simulink model "TCMSSystem"  (R2019b)
settings: configuration reference "ConfigSet_TCMSSystem_Reference" (kept outside this file)
model workspace (MAT data in the model file):
  Prm_TCMSSystem : Simulink.Parameter (value not decoded)
  SampleTime = 0.05
symbols that are objects in the model workspace (value not decoded): Prm_TCMSSystem
undefined symbols (not defined in the file): ADDIntervention, AK1Status, AK2Status, AKContactorStatus, AllDoorsClosed, AllLeftDoorsClosed, AllRightDoorsClosed, APS1Fault, APS1Isolated, APS1OutputVoltage, APS1Status, APS2Fault, APS2Isolated, APS2OutputVoltage, APS2Status, APSKAKContactor, ASCOEnd1, ASCOEnd2, ATBMode, ATCBypassMode, ATCStatusNotOK, ATOMode, ATPLowSpeedCutoutStatus, ATPMode, AuxCompressor, BatteryCurrent, BatteryIsolationContactor, BatteryTemperature, BatteryVoltage, BCG1Fault, BCG1Isolated, BCG1IsolationFailed, BCG1OutputCurrent, BCG1Status, BCG2Fault, BCG2Isolated, BCG2OutputCurrent, BCG2Status, BCGOutputVoltage, BECU1AxleLockedWheelSet1, BECU2AxleLockedWheelSet2, BECUFaulty, BECUMajorFault, BECUMinorFault, BECUStatus, BIC1Inside, BIC1Outside, BIC2Inside, BIC2Outside, Bogie, Bogie1WSPStatus, Bogie2WSPStatus, BogieFaulty, BogieIsolationStatus, BogieSupportedMass, BrakeCylinderPressureGauge, BrakeLoopCBTripped, BrakeLoopOpenTL, BrakeTrainLineStatus, BrakingDemand ... (+215)
libraries: TimersLib x257, simulink x137, LatchesLib x42, VectorOperationsLib x15, TestBenchLib x12, MathOperationsLib x2, FiltersLib x1
(part 11 of 16)

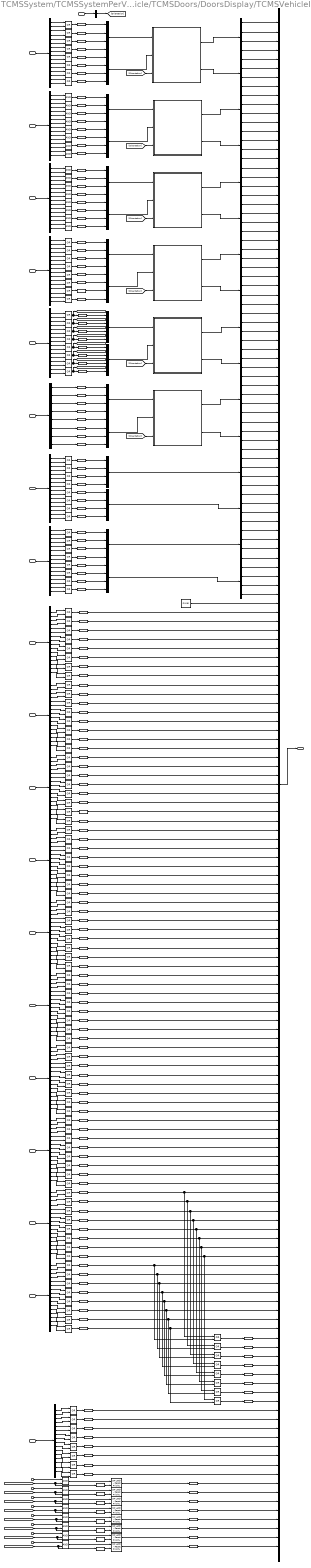
== system TCMSSystem/TCMSSystemPerVehicle/EnabledTCMSVehicle/TCMSDoors/DoorsDisplay/TCMSVehicleInfo/Subsystem1 ==
  CommonVehicleConfig : Inport
  DoorOpenStatus : Inport  Port=2
  DoorEmergencyReleasedStatus : Inport  Port=3
  DoorIsolatedStatus : Inport  Port=4
  DoorFaultStatus : Inport  Port=5
  DoorLockedStatus : Inport  Port=6
  DoorCloseObstruction : Inport  Port=7
  DoorOpenObstruction : Inport  Port=8
  DoorMotorCircuitFailure : Inport  Port=9
  DoorFailedToLock : Inport  Port=10
  DoorFailedToUnlock : Inport  Port=11
  DoorUnexpectedUnlocking : Inport  Port=12
  DCUFailure : Inport  Port=13
  DCSRFailure : Inport  Port=14
  DCSLFailure : Inport  Port=15
  DLSRFailure : Inport  Port=16
  DLSLFailure : Inport  Port=17
  DoorMajorFault : Inport  Port=18
  UnexpectedDoorOpeningDetectedByCC : Inport  Port=19
  DCUPower : Inport  Port=20
  In Bus Element : Inport  Port=21  PortName=InputControlStates  Element=LeftDoor1EED
  In Bus Element2 : Inport  Port=21  PortName=InputControlStates  Element=LeftDoor2EED
  In Bus Element3 : Inport  Port=21  PortName=InputControlStates  Element=LeftDoor3EED
  In Bus Element4 : Inport  Port=21  PortName=InputControlStates  Element=LeftDoor4EED
  In Bus Element5 : Inport  Port=21  PortName=InputControlStates  Element=RightDoor1EED
  In Bus Element6 : Inport  Port=21  PortName=InputControlStates  Element=RightDoor2EED
  In Bus Element7 : Inport  Port=21  PortName=InputControlStates  Element=RightDoor3EED
  In Bus Element8 : Inport  Port=21  PortName=InputControlStates  Element=RightDoor4EED
  Bus Creator : BusCreator  Inputs=169  OutDataTypeStr=Bus: BD_TCMSSystem_Out_Vehicle_Display_DoorSystem_Door  NonVirtualBus=on
  Bus Selector : BusSelector  OutputSignals=Orientation
  Data Type Conversion{1..168} (168 alike) : DataTypeConversion
  Demux : Demux  Outputs=8
  Demux{1..4,17,22,24..35} (18 alike) : Demux  Outputs=16
  Demux{5..16,19..21,23} (16 alike) : Demux
  Detect Decrease{,1..7} (8 alike) : simulink/Logic and Bit Operations/Detect Decrease  vinit=0.0  OutDataTypeStr=boolean
  FIXME2 : TestBenchLib/FIXME
      settings: SourceProductName=Sydac Utilities
  For Each Subsystem1 : Subsystem  TreatAsAtomicUnit=on
  For Each Subsystem2 : Subsystem  TreatAsAtomicUnit=on
  For Each Subsystem3 : Subsystem  TreatAsAtomicUnit=on
  For Each Subsystem4 : Subsystem  TreatAsAtomicUnit=on
  For Each Subsystem5 : Subsystem  TreatAsAtomicUnit=on
  For Each Subsystem6 : Subsystem  TreatAsAtomicUnit=on
  OR{,1..15,24..39,48..135,144..159} (136 alike) : Logic  Operator=OR  AllPortsSameDT=off  OutDataTypeStr=boolean
  OR{16..23,40..47,136..143} (24 alike) : Logic  AllPortsSameDT=off  OutDataTypeStr=boolean
  SR Latch - Reset Priority{,1..7} (8 alike) : LatchesLib/SR Latch - Reset Priority  initial_condition=0
      settings: SourceProductName=Latches
  Vector Concatenate{,1..15} (16 alike) : Concatenate  NumInputs=4
  TCMSDoorStatus : Outport
  wires:
  Bus Creator/1 -> TCMSDoorStatus/1
  Demux13/3 -> Bus Creator/39  "DoorB3EmergencyReleased"
  Demux14/4 -> Bus Creator/36  "DoorA4EmergencyReleased"
  Demux14/2 -> Bus Creator/34  "DoorA2EmergencyReleased"
  Demux13/2 -> Bus Creator/38  "DoorB2EmergencyReleased"
  Demux14/1 -> Bus Creator/33  "DoorA1EmergencyReleased"
  Demux13/1 -> Bus Creator/37  "DoorB1EmergencyReleased"
  Demux13/4 -> Bus Creator/40  "DoorB4EmergencyReleased"
  Demux14/3 -> Bus Creator/35  "DoorA3EmergencyReleased"
  Demux10/4 -> Bus Creator/24  "DoorB4Isolated"
  Demux10/3 -> Bus Creator/23  "DoorB3Isolated"
  Demux10/2 -> Bus Creator/22  "DoorB2Isolated"
  Demux10/1 -> Bus Creator/21  "DoorB1Isolated"
  Demux9/3 -> Bus Creator/19  "DoorA3Isolated"
  Demux9/4 -> Bus Creator/20  "DoorA4Isolated"
  Demux9/1 -> Bus Creator/17  "DoorA1Isolated"
  Demux9/2 -> Bus Creator/18  "DoorA2Isolated"
  Demux11/4 -> Bus Creator/32  "DoorB4Fault"
  Demux12/1 -> Bus Creator/25  "DoorA1Fault"
  Demux12/4 -> Bus Creator/28  "DoorA4Fault"
  Demux12/3 -> Bus Creator/27  "DoorA3Fault"
  Demux12/2 -> Bus Creator/26  "DoorA2Fault"
  Demux11/3 -> Bus Creator/31  "DoorB3Fault"
  Demux11/1 -> Bus Creator/29  "DoorB1Fault"
  Demux11/2 -> Bus Creator/30  "DoorB2Fault"
  CommonVehicleConfig/1 -> Bus Selector/1
  Demux7/1 -> Bus Creator/9  "DoorA1Locked"
  Demux7/2 -> Bus Creator/10  "DoorA2Locked"
  Demux7/3 -> Bus Creator/11  "DoorA3Locked"
  Demux7/4 -> Bus Creator/12  "DoorA4Locked"
  Demux8/1 -> Bus Creator/13  "DoorB1Locked"
  Demux8/2 -> Bus Creator/14  "DoorB2Locked"
  Demux8/3 -> Bus Creator/15  "DoorB3Locked"
  Demux8/4 -> Bus Creator/16  "DoorB4Locked"
  Demux5/1 -> Bus Creator/1  "DoorA1Open"
  Demux5/2 -> Bus Creator/2  "DoorA2Open"
  Demux5/3 -> Bus Creator/3  "DoorA3Open"
  Demux5/4 -> Bus Creator/4  "DoorA4Open"
  Demux6/1 -> Bus Creator/5  "DoorB1Open"
  Demux6/2 -> Bus Creator/6  "DoorB2Open"
  Demux6/3 -> Bus Creator/7  "DoorB3Open"
  Demux6/4 -> Bus Creator/8  "DoorB4Open"
  Data Type Conversion152/1 -> Vector Concatenate/1  "DoorA1Open"
  Data Type Conversion153/1 -> Vector Concatenate/2  "DoorA2Open"
  Data Type Conversion146/1 -> Vector Concatenate/3  "DoorA3Open"
  Data Type Conversion147/1 -> Vector Concatenate/4  "DoorA4Open"
  Data Type Conversion150/1 -> Vector Concatenate1/1  "DoorB1Open"
  Data Type Conversion151/1 -> Vector Concatenate1/2  "DoorB2Open"
  Data Type Conversion148/1 -> Vector Concatenate1/3  "DoorB3Open"
  Data Type Conversion149/1 -> Vector Concatenate1/4  "DoorB4Open"
  Bus Selector/1 -> [Orientation]  "<Orientation>"
  Data Type Conversion98/1 -> Vector Concatenate2/1  "DoorA1Locked"
  Data Type Conversion99/1 -> Vector Concatenate2/2  "DoorA2Locked"
  Data Type Conversion100/1 -> Vector Concatenate2/3  "DoorA3Locked"
  Data Type Conversion101/1 -> Vector Concatenate2/4  "DoorA4Locked"
  Data Type Conversion104/1 -> Vector Concatenate3/1  "DoorB1Locked"
  Data Type Conversion105/1 -> Vector Concatenate3/2  "DoorB2Locked"
  Data Type Conversion102/1 -> Vector Concatenate3/3  "DoorB3Locked"
  Data Type Conversion103/1 -> Vector Concatenate3/4  "DoorB4Locked"
  Data Type Conversion144/1 -> Vector Concatenate4/1  "DoorA1Isolated"
  Data Type Conversion145/1 -> Vector Concatenate4/2  "DoorA2Isolated"
  Data Type Conversion138/1 -> Vector Concatenate4/3  "DoorA3Isolated"
  Data Type Conversion139/1 -> Vector Concatenate4/4  "DoorA4Isolated"
  Data Type Conversion142/1 -> Vector Concatenate5/1  "DoorB1Isolated"
  Data Type Conversion143/1 -> Vector Concatenate5/2  "DoorB2Isolated"
  Data Type Conversion140/1 -> Vector Concatenate5/3  "DoorB3Isolated"
  Data Type Conversion141/1 -> Vector Concatenate5/4  "DoorB4Isolated"
  Data Type Conversion136/1 -> Vector Concatenate6/1  "DoorA1Fault"
  Data Type Conversion137/1 -> Vector Concatenate6/2  "DoorA2Fault"
  Data Type Conversion130/1 -> Vector Concatenate6/3  "DoorA3Fault"
  Data Type Conversion131/1 -> Vector Concatenate6/4  "DoorA4Fault"
  Data Type Conversion134/1 -> Vector Concatenate7/1  "DoorB1Fault"
  Data Type Conversion135/1 -> Vector Concatenate7/2  "DoorB2Fault"
  Data Type Conversion132/1 -> Vector Concatenate7/3  "DoorB3Fault"
  Data Type Conversion133/1 -> Vector Concatenate7/4  "DoorB4Fault"
  Data Type Conversion128/1 -> Vector Concatenate8/1  "DoorA1EmergencyReleased"
  Data Type Conversion129/1 -> Vector Concatenate8/2  "DoorA2EmergencyReleased"
  Data Type Conversion122/1 -> Vector Concatenate8/3  "DoorA3EmergencyReleased"
  Data Type Conversion123/1 -> Vector Concatenate8/4  "DoorA4EmergencyReleased"
  Data Type Conversion126/1 -> Vector Concatenate9/1  "DoorB1EmergencyReleased"
  Data Type Conversion127/1 -> Vector Concatenate9/2  "DoorB2EmergencyReleased"
  Data Type Conversion124/1 -> Vector Concatenate9/3  "DoorB3EmergencyReleased"
  Data Type Conversion125/1 -> Vector Concatenate9/4  "DoorB4EmergencyReleased"
  Demux16/3 -> Bus Creator/43  "DCU3Status"
  Demux15/4 -> Bus Creator/48  "DCU8Status"
  Demux15/1 -> Bus Creator/45  "DCU5Status"
  Demux15/2 -> Bus Creator/46  "DCU6Status"
  Demux16/2 -> Bus Creator/42  "DCU2Status"
  Demux16/4 -> Bus Creator/44  "DCU4Status"
  Demux15/3 -> Bus Creator/47  "DCU7Status"
  Demux16/1 -> Bus Creator/41  "DCU1Status"
  For Each Subsystem2/1(WireState1) -> Demux5/1
  For Each Subsystem2/2(WireState2) -> Demux6/1
  Vector Concatenate1/1 -> For Each Subsystem2/2(Source2)
  Vector Concatenate/1 -> For Each Subsystem2/1(Source1)
  [Orientation] -> For Each Subsystem2/3(Orientation)
  [Orientation] -> For Each Subsystem3/3(Orientation)
  Vector Concatenate2/1 -> For Each Subsystem3/1(Source1)
  Vector Concatenate3/1 -> For Each Subsystem3/2(Source2)
  For Each Subsystem3/2(WireState2) -> Demux8/1
  For Each Subsystem3/1(WireState1) -> Demux7/1
  For Each Subsystem4/1(WireState1) -> Demux9/1
  For Each Subsystem4/2(WireState2) -> Demux10/1
  Vector Concatenate5/1 -> For Each Subsystem4/2(Source2)
  Vector Concatenate4/1 -> For Each Subsystem4/1(Source1)
  [Orientation] -> For Each Subsystem4/3(Orientation)
  [Orientation] -> For Each Subsystem5/3(Orientation)
  Vector Concatenate8/1 -> For Each Subsystem5/1(Source1)
  Vector Concatenate9/1 -> For Each Subsystem5/2(Source2)
  For Each Subsystem5/2(WireState2) -> Demux13/1
  For Each Subsystem5/1(WireState1) -> Demux14/1
  [Orientation] -> For Each Subsystem1/3(Orientation)
  Vector Concatenate6/1 -> For Each Subsystem1/1(Source1)
  Vector Concatenate7/1 -> For Each Subsystem1/2(Source2)
  For Each Subsystem1/2(WireState2) -> Demux11/1
  For Each Subsystem1/1(WireState1) -> Demux12/1
  Data Type Conversion17/1 -> Bus Creator/73  "DoorB4MotorCircuitFailure"
  Data Type Conversion15/1 -> Bus Creator/71  "DoorB2MotorCircuitFailure"
  Data Type Conversion16/1 -> Bus Creator/72  "DoorB3MotorCircuitFailure"
  Demux21/4 -> Bus Creator/52  "DoorA4CloseObstruction"
  Vector Concatenate12/1 -> Demux23/1
  Vector Concatenate10/1 -> Demux21/1
  Vector Concatenate11/1 -> Demux20/1
  Demux23/2 -> Bus Creator/58  "DoorA2OpenObstruction"
  Data Type Conversion110/1 -> Vector Concatenate13/1  "DoorB1OpenObstruction"
  Demux19/3 -> Bus Creator/63  "DoorB3OpenObstruction"
  Data Type Conversion109/1 -> Vector Concatenate13/4  "DoorB4OpenObstruction"
  Data Type Conversion112/1 -> Vector Concatenate12/1  "DoorA1OpenObstruction"
  Data Type Conversion108/1 -> Vector Concatenate13/3  "DoorB3OpenObstruction"
  Demux19/1 -> Bus Creator/61  "DoorB1OpenObstruction"
  Data Type Conversion111/1 -> Vector Concatenate13/2  "DoorB2OpenObstruction"
  Data Type Conversion121/1 -> Vector Concatenate10/2  "DoorA2CloseObstruction"
  Demux21/1 -> Bus Creator/49  "DoorA1CloseObstruction"
  Data Type Conversion115/1 -> Vector Concatenate10/4  "DoorA4CloseObstruction"
  Demux21/2 -> Bus Creator/50  "DoorA2CloseObstruction"
  Demux20/2 -> Bus Creator/54  "DoorB2CloseObstruction"
  Demux21/3 -> Bus Creator/51  "DoorA3CloseObstruction"
  Demux23/1 -> Bus Creator/57  "DoorA1OpenObstruction"
  Data Type Conversion114/1 -> Vector Concatenate10/3  "DoorA3CloseObstruction"
  Vector Concatenate13/1 -> Demux19/1
  Data Type Conversion92/1 -> Bus Creator/76  "DoorA3FailedToLock"
  Data Type Conversion96/1 -> Bus Creator/80  "DoorB3FailedToLock"
  Data Type Conversion90/1 -> Bus Creator/74  "DoorA1FailedToLock"
  Data Type Conversion97/1 -> Bus Creator/81  "DoorB4FailedToLock"
  Data Type Conversion91/1 -> Bus Creator/75  "DoorA2FailedToLock"
  Data Type Conversion94/1 -> Bus Creator/78  "DoorB1FailedToLock"
  Data Type Conversion62/1 -> Bus Creator/110  "DoorB1DCSLFailure"
  Data Type Conversion95/1 -> Bus Creator/79  "DoorB2FailedToLock"
  Data Type Conversion60/1 -> Bus Creator/108  "DoorA3DCSLFailure"
  Data Type Conversion52/1 -> Bus Creator/116  "DoorA3DLSRFailure"
  Data Type Conversion50/1 -> Bus Creator/114  "DoorA1DLSRFailure"
  Data Type Conversion63/1 -> Bus Creator/111  "DoorB2DCSLFailure"
  Data Type Conversion51/1 -> Bus Creator/115  "DoorA2DLSRFailure"
  Data Type Conversion61/1 -> Bus Creator/109  "DoorA4DCSLFailure"
  Data Type Conversion65/1 -> Bus Creator/113  "DoorB4DCSLFailure"
  Data Type Conversion87/1 -> Bus Creator/87  "DoorB2FailedToUnlock"
  Data Type Conversion89/1 -> Bus Creator/89  "DoorB4FailedToUnlock"
  Data Type Conversion86/1 -> Bus Creator/86  "DoorB1FailedToUnlock"
  Data Type Conversion88/1 -> Bus Creator/88  "DoorB3FailedToUnlock"
  Data Type Conversion84/1 -> Bus Creator/84  "DoorA3FailedToUnlock"
  Data Type Conversion83/1 -> Bus Creator/83  "DoorA2FailedToUnlock"
  Data Type Conversion82/1 -> Bus Creator/82  "DoorA1FailedToUnlock"
  Data Type Conversion117/1 -> Vector Concatenate11/4  "DoorB4CloseObstruction"
  Data Type Conversion85/1 -> Bus Creator/85  "DoorA4FailedToUnlock"
  Data Type Conversion113/1 -> Vector Concatenate12/2  "DoorA2OpenObstruction"
  Data Type Conversion13/1 -> Bus Creator/69  "DoorA4MotorCircuitFailure"
  Data Type Conversion120/1 -> Vector Concatenate10/1  "DoorA1CloseObstruction"
  Data Type Conversion14/1 -> Bus Creator/70  "DoorB1MotorCircuitFailure"
  Data Type Conversion11/1 -> Bus Creator/67  "DoorA2MotorCircuitFailure"
  Demux20/4 -> Bus Creator/56  "DoorB4CloseObstruction"
  Data Type Conversion79/1 -> Bus Creator/95  "DoorB2UnexpectedUnlocking"
  Data Type Conversion75/1 -> Bus Creator/91  "DoorA2UnexpectedUnlocking"
  Data Type Conversion80/1 -> Bus Creator/96  "DoorB3UnexpectedUnlocking"
  Data Type Conversion119/1 -> Vector Concatenate11/2  "DoorB2CloseObstruction"
  Data Type Conversion78/1 -> Bus Creator/94  "DoorB1UnexpectedUnlocking"
  Data Type Conversion28/1 -> OR2/2, Bus Creator/140  "DoorA3DCUFailure"
  Data Type Conversion81/1 -> Bus Creator/97  "DoorB4UnexpectedUnlocking"
  Demux23/4 -> Bus Creator/60  "DoorA4OpenObstruction"
  Demux20/3 -> Bus Creator/55  "DoorB3CloseObstruction"
  Data Type Conversion106/1 -> Vector Concatenate12/3  "DoorA3OpenObstruction"
  Demux19/2 -> Bus Creator/62  "DoorB2OpenObstruction"
  Data Type Conversion26/1 -> OR/2, Bus Creator/138  "DoorA1DCUFailure"
  Data Type Conversion31/1 -> OR5/2, Bus Creator/143  "DoorB2DCUFailure"
  Data Type Conversion27/1 -> OR1/2, Bus Creator/139  "DoorA2DCUFailure"
  Data Type Conversion32/1 -> OR6/2, Bus Creator/144  "DoorB3DCUFailure"
  Data Type Conversion30/1 -> OR4/2, Bus Creator/142  "DoorB1DCUFailure"
  Data Type Conversion54/1 -> Bus Creator/118  "DoorB1DLSRFailure"
  Data Type Conversion34/1 -> OR/1, Bus Creator/130  "DoorA1DoorMajorFault"
  Data Type Conversion56/1 -> Bus Creator/120  "DoorB3DLSRFailure"
  Data Type Conversion107/1 -> Vector Concatenate12/4  "DoorA4OpenObstruction"
  Data Type Conversion40/1 -> OR6/1, Bus Creator/136  "DoorB3DoorMajorFault"
  Data Type Conversion76/1 -> Bus Creator/92  "DoorA3UnexpectedUnlocking"
  Data Type Conversion58/1 -> Bus Creator/106  "DoorA1DCSLFailure"
  Data Type Conversion53/1 -> Bus Creator/117  "DoorA4DLSRFailure"
  Data Type Conversion33/1 -> OR7/2, Bus Creator/145  "DoorB4DCUFailure"
  Data Type Conversion72/1 -> Bus Creator/104  "DoorB3DCSRFailure"
  Data Type Conversion93/1 -> Bus Creator/77  "DoorA4FailedToLock"
  Data Type Conversion64/1 -> Bus Creator/112  "DoorB3DCSLFailure"
  Data Type Conversion71/1 -> Bus Creator/103  "DoorB2DCSRFailure"
  Data Type Conversion70/1 -> Bus Creator/102  "DoorB1DCSRFailure"
  Data Type Conversion74/1 -> Bus Creator/90  "DoorA1UnexpectedUnlocking"
  Data Type Conversion73/1 -> Bus Creator/105  "DoorB4DCSRFailure"
  Demux23/3 -> Bus Creator/59  "DoorA3OpenObstruction"
  Data Type Conversion68/1 -> Bus Creator/100  "DoorA3DCSRFailure"
  Data Type Conversion12/1 -> Bus Creator/68  "DoorA3MotorCircuitFailure"
  Data Type Conversion67/1 -> Bus Creator/99  "DoorA2DCSRFailure"
  Data Type Conversion66/1 -> Bus Creator/98  "DoorA1DCSRFailure"
  Data Type Conversion38/1 -> OR4/1, Bus Creator/134  "DoorB1DoorMajorFault"
  Data Type Conversion44/1 -> Bus Creator/124  "DoorA3DLSLFailure"
  Data Type Conversion48/1 -> Bus Creator/128  "DoorB3DLSLFailure"
  FIXME2/1 -> Bus Creator/65  "DoorA1OpenDummyForLeaf"
  Data Type Conversion35/1 -> OR1/1, Bus Creator/131  "DoorA2DoorMajorFault"
  Data Type Conversion10/1 -> Bus Creator/66  "DoorA1MotorCircuitFailure"
  Data Type Conversion45/1 -> Bus Creator/125  "DoorA4DLSLFailure"
  Data Type Conversion118/1 -> Vector Concatenate11/1  "DoorB1CloseObstruction"
  Data Type Conversion46/1 -> Bus Creator/126  "DoorB1DLSLFailure"
  Demux19/4 -> Bus Creator/64  "DoorB4OpenObstruction"
  Data Type Conversion55/1 -> Bus Creator/119  "DoorB2DLSRFailure"
  Data Type Conversion37/1 -> OR3/1, Bus Creator/133  "DoorA4DoorMajorFault"
  Demux20/1 -> Bus Creator/53  "DoorB1CloseObstruction"
  Data Type Conversion49/1 -> Bus Creator/129  "DoorB4DLSLFailure"
  Data Type Conversion43/1 -> Bus Creator/123  "DoorA2DLSLFailure"
  Data Type Conversion42/1 -> Bus Creator/122  "DoorA1DLSLFailure"
  Data Type Conversion69/1 -> Bus Creator/101  "DoorA4DCSRFailure"
  Data Type Conversion36/1 -> OR2/1, Bus Creator/132  "DoorA3DoorMajorFault"
  Data Type Conversion59/1 -> Bus Creator/107  "DoorA2DCSLFailure"
  Data Type Conversion39/1 -> OR5/1, Bus Creator/135  "DoorB2DoorMajorFault"
  Data Type Conversion41/1 -> OR7/1, Bus Creator/137  "DoorB4DoorMajorFault"
  Data Type Conversion77/1 -> Bus Creator/93  "DoorA4UnexpectedUnlocking"
  Data Type Conversion47/1 -> Bus Creator/127  "DoorB2DLSLFailure"
  Data Type Conversion29/1 -> OR3/2, Bus Creator/141  "DoorA4DCUFailure"
  Data Type Conversion116/1 -> Vector Concatenate11/3  "DoorB3CloseObstruction"
  Data Type Conversion57/1 -> Bus Creator/121  "DoorB4DLSRFailure"
  OR2/1 -> Data Type Conversion4/1
  OR/1 -> Data Type Conversion2/1
  OR6/1 -> Data Type Conversion8/1
  OR1/1 -> Data Type Conversion3/1
  OR4/1 -> Data Type Conversion6/1
  OR3/1 -> Data Type Conversion5/1
  OR7/1 -> Data Type Conversion9/1
  OR5/1 -> Data Type Conversion7/1
  Data Type Conversion2/1 -> Bus Creator/146  "DCU1Fault"
  Data Type Conversion3/1 -> Bus Creator/147  "DCU2Fault"
  Data Type Conversion4/1 -> Bus Creator/148  "DCU3Fault"
  Data Type Conversion5/1 -> Bus Creator/149  "DCU4Fault"
  Data Type Conversion6/1 -> Bus Creator/150  "DCU5Fault"
  Data Type Conversion7/1 -> Bus Creator/151  "DCU6Fault"
  Data Type Conversion8/1 -> Bus Creator/152  "DCU7Fault"
  Data Type Conversion9/1 -> Bus Creator/153  "DCU8Fault"
  Data Type Conversion18/1 -> Bus Creator/154  "DoorA1UnexpectedOpen"
  Data Type Conversion19/1 -> Bus Creator/155  "DoorA2UnexpectedOpen"
  Data Type Conversion20/1 -> Bus Creator/156  "DoorA3UnexpectedOpen"
  Data Type Conversion21/1 -> Bus Creator/157  "DoorA4UnexpectedOpen"
  Data Type Conversion22/1 -> Bus Creator/158  "DoorB1UnexpectedOpen"
  Data Type Conversion23/1 -> Bus Creator/159  "DoorB2UnexpectedOpen"
  Data Type Conversion24/1 -> Bus Creator/160  "DoorB3UnexpectedOpen"
  Data Type Conversion25/1 -> Bus Creator/161  "DoorB4UnexpectedOpen"
  UnexpectedDoorOpeningDetectedByCC/1 -> Demux34/1  "DCU8Fault"
  Demux35/8 -> OR157/2
  Demux35/4 -> OR155/2
  Demux35/2 -> OR154/2
  Demux35/3 -> OR155/1
  Demux35/16 -> OR159/2
  Demux35/12 -> OR153/2
  Demux35/6 -> OR156/2
  Demux35/9 -> OR152/1
  Demux35/10 -> OR152/2
  Demux35/15 -> OR159/1
  Demux35/1 -> OR154/1
  Demux35/11 -> OR153/1
  Demux35/7 -> OR157/1
  Demux35/13 -> OR158/1
  Demux35/5 -> OR156/1
  Demux35/14 -> OR158/2
  OR154/1 -> Data Type Conversion10/1
  OR155/1 -> Data Type Conversion11/1
  OR157/1 -> Data Type Conversion13/1
  OR156/1 -> Data Type Conversion12/1
  OR158/1 -> Data Type Conversion16/1
  OR159/1 -> Data Type Conversion17/1
  OR153/1 -> Data Type Conversion15/1
  OR152/1 -> Data Type Conversion14/1
  OR144/1 -> Data Type Conversion22/1
  OR145/1 -> Data Type Conversion23/1
  OR151/1 -> Data Type Conversion25/1
  OR150/1 -> Data Type Conversion24/1
  OR148/1 -> Data Type Conversion20/1
  OR149/1 -> Data Type Conversion21/1
  OR147/1 -> Data Type Conversion19/1
  OR146/1 -> Data Type Conversion18/1
  Demux34/14 -> OR150/2
  Demux34/5 -> OR148/1
  Demux34/13 -> OR150/1
  Demux34/7 -> OR149/1
  Demux34/11 -> OR145/1
  Demux34/1 -> OR146/1
  Demux34/15 -> OR151/1
  Demux34/10 -> OR144/2
  Demux34/9 -> OR144/1
  Demux34/6 -> OR148/2
  Demux34/12 -> OR145/2
  Demux34/16 -> OR151/2
  Demux34/3 -> OR147/1
  Demux34/2 -> OR146/2
  Demux34/4 -> OR147/2
  Demux34/8 -> OR149/2
  OR64/1 -> Data Type Conversion30/1
  OR65/1 -> Data Type Conversion31/1
  OR71/1 -> Data Type Conversion33/1
  OR70/1 -> Data Type Conversion32/1
  OR68/1 -> Data Type Conversion28/1
  OR69/1 -> Data Type Conversion29/1
  OR67/1 -> Data Type Conversion27/1
  OR66/1 -> Data Type Conversion26/1
  Demux17/14 -> OR70/2
  Demux17/5 -> OR68/1
  Demux17/13 -> OR70/1
  Demux17/7 -> OR69/1
  Demux17/11 -> OR65/1
  Demux17/1 -> OR66/1
  Demux17/15 -> OR71/1
  Demux17/10 -> OR64/2
  Demux17/9 -> OR64/1
  Demux17/6 -> OR68/2
  Demux17/12 -> OR65/2
  Demux17/16 -> OR71/2
  Demux17/3 -> OR67/1
  Demux17/2 -> OR66/2
  Demux17/4 -> OR67/2
  Demux17/8 -> OR69/2
  DCUFailure/1 -> Demux17/1
  OR72/1 -> Data Type Conversion38/1
  OR73/1 -> Data Type Conversion39/1
  OR79/1 -> Data Type Conversion41/1
  OR78/1 -> Data Type Conversion40/1
  OR76/1 -> Data Type Conversion36/1
  OR77/1 -> Data Type Conversion37/1
  OR75/1 -> Data Type Conversion35/1
  OR74/1 -> Data Type Conversion34/1
  Demux25/14 -> OR78/2
  Demux25/5 -> OR76/1
  Demux25/13 -> OR78/1
  Demux25/7 -> OR77/1
  Demux25/11 -> OR73/1
  Demux25/1 -> OR74/1
  Demux25/15 -> OR79/1
  Demux25/10 -> OR72/2
  Demux25/9 -> OR72/1
  Demux25/6 -> OR76/2
  Demux25/12 -> OR73/2
  Demux25/16 -> OR79/2
  Demux25/3 -> OR75/1
  Demux25/2 -> OR74/2
  Demux25/4 -> OR75/2
  Demux25/8 -> OR77/2
  DoorMajorFault/1 -> Demux25/1
  OR80/1 -> Data Type Conversion46/1
  OR81/1 -> Data Type Conversion47/1
  OR87/1 -> Data Type Conversion49/1
  OR86/1 -> Data Type Conversion48/1
  OR84/1 -> Data Type Conversion44/1
  OR85/1 -> Data Type Conversion45/1
  OR83/1 -> Data Type Conversion43/1
  OR82/1 -> Data Type Conversion42/1
  Demux26/14 -> OR86/2
  Demux26/5 -> OR84/1
  Demux26/13 -> OR86/1
  Demux26/7 -> OR85/1
  Demux26/11 -> OR81/1
  Demux26/1 -> OR82/1
  Demux26/15 -> OR87/1
  Demux26/10 -> OR80/2
  Demux26/9 -> OR80/1
  Demux26/6 -> OR84/2
  Demux26/12 -> OR81/2
  Demux26/16 -> OR87/2
  Demux26/3 -> OR83/1
  Demux26/2 -> OR82/2
  Demux26/4 -> OR83/2
  Demux26/8 -> OR85/2
  DLSLFailure/1 -> Demux26/1
  OR88/1 -> Data Type Conversion54/1
  OR89/1 -> Data Type Conversion55/1
  OR95/1 -> Data Type Conversion57/1
  OR94/1 -> Data Type Conversion56/1
  OR92/1 -> Data Type Conversion52/1
  OR93/1 -> Data Type Conversion53/1
  OR91/1 -> Data Type Conversion51/1
  OR90/1 -> Data Type Conversion50/1
  Demux27/14 -> OR94/2
  Demux27/5 -> OR92/1
  Demux27/13 -> OR94/1
  Demux27/7 -> OR93/1
  Demux27/11 -> OR89/1
  Demux27/1 -> OR90/1
  Demux27/15 -> OR95/1
  Demux27/10 -> OR88/2
  Demux27/9 -> OR88/1
  Demux27/6 -> OR92/2
  Demux27/12 -> OR89/2
  Demux27/16 -> OR95/2
  Demux27/3 -> OR91/1
  Demux27/2 -> OR90/2
  Demux27/4 -> OR91/2
  Demux27/8 -> OR93/2
  DLSRFailure/1 -> Demux27/1
  OR96/1 -> Data Type Conversion62/1
  OR97/1 -> Data Type Conversion63/1
  OR103/1 -> Data Type Conversion65/1
  OR102/1 -> Data Type Conversion64/1
  OR100/1 -> Data Type Conversion60/1
  OR101/1 -> Data Type Conversion61/1
  OR99/1 -> Data Type Conversion59/1
  OR98/1 -> Data Type Conversion58/1
  Demux28/14 -> OR102/2
  Demux28/5 -> OR100/1
  Demux28/13 -> OR102/1
  Demux28/7 -> OR101/1
  Demux28/11 -> OR97/1
  Demux28/1 -> OR98/1
  Demux28/15 -> OR103/1
  Demux28/10 -> OR96/2
  Demux28/9 -> OR96/1
  Demux28/6 -> OR100/2
  Demux28/12 -> OR97/2
  Demux28/16 -> OR103/2
  Demux28/3 -> OR99/1
  Demux28/2 -> OR98/2
  Demux28/4 -> OR99/2
  Demux28/8 -> OR101/2
  DCSLFailure/1 -> Demux28/1
  OR104/1 -> Data Type Conversion70/1
  OR105/1 -> Data Type Conversion71/1
  OR111/1 -> Data Type Conversion73/1
  OR110/1 -> Data Type Conversion72/1
  OR108/1 -> Data Type Conversion68/1
  OR109/1 -> Data Type Conversion69/1
  OR107/1 -> Data Type Conversion67/1
  OR106/1 -> Data Type Conversion66/1
  Demux29/14 -> OR110/2
  Demux29/5 -> OR108/1
  Demux29/13 -> OR110/1
  Demux29/7 -> OR109/1
  Demux29/11 -> OR105/1
  Demux29/1 -> OR106/1
  Demux29/15 -> OR111/1
  Demux29/10 -> OR104/2
  Demux29/9 -> OR104/1
  Demux29/6 -> OR108/2
  Demux29/12 -> OR105/2
  Demux29/16 -> OR111/2
  Demux29/3 -> OR107/1
  Demux29/2 -> OR106/2
  Demux29/4 -> OR107/2
  Demux29/8 -> OR109/2
  OR112/1 -> Data Type Conversion78/1
  OR113/1 -> Data Type Conversion79/1
  OR119/1 -> Data Type Conversion81/1
  OR118/1 -> Data Type Conversion80/1
  OR116/1 -> Data Type Conversion76/1
  OR117/1 -> Data Type Conversion77/1
  OR115/1 -> Data Type Conversion75/1
  OR114/1 -> Data Type Conversion74/1
  Demux30/14 -> OR118/2
  Demux30/5 -> OR116/1
  Demux30/13 -> OR118/1
  Demux30/7 -> OR117/1
  Demux30/11 -> OR113/1
  Demux30/1 -> OR114/1
  Demux30/15 -> OR119/1
  Demux30/10 -> OR112/2
  Demux30/9 -> OR112/1
  Demux30/6 -> OR116/2
  Demux30/12 -> OR113/2
  Demux30/16 -> OR119/2
  Demux30/3 -> OR115/1
  Demux30/2 -> OR114/2
  Demux30/4 -> OR115/2
  Demux30/8 -> OR117/2
  OR120/1 -> Data Type Conversion86/1
  OR121/1 -> Data Type Conversion87/1
  OR127/1 -> Data Type Conversion89/1
  OR126/1 -> Data Type Conversion88/1
  OR124/1 -> Data Type Conversion84/1
  OR125/1 -> Data Type Conversion85/1
  OR123/1 -> Data Type Conversion83/1
  OR122/1 -> Data Type Conversion82/1
  Demux31/14 -> OR126/2
  Demux31/5 -> OR124/1
  Demux31/13 -> OR126/1
  Demux31/7 -> OR125/1
  Demux31/11 -> OR121/1
  Demux31/1 -> OR122/1
  Demux31/15 -> OR127/1
  Demux31/10 -> OR120/2
  Demux31/9 -> OR120/1
  Demux31/6 -> OR124/2
  Demux31/12 -> OR121/2
  Demux31/16 -> OR127/2
  Demux31/3 -> OR123/1
  Demux31/2 -> OR122/2
  Demux31/4 -> OR123/2
  Demux31/8 -> OR125/2
  OR128/1 -> Data Type Conversion94/1
  OR129/1 -> Data Type Conversion95/1
  OR135/1 -> Data Type Conversion97/1
  OR134/1 -> Data Type Conversion96/1
  OR132/1 -> Data Type Conversion92/1
  OR133/1 -> Data Type Conversion93/1
  OR131/1 -> Data Type Conversion91/1
  OR130/1 -> Data Type Conversion90/1
  Demux32/14 -> OR134/2
  Demux32/5 -> OR132/1
  Demux32/13 -> OR134/1
  Demux32/7 -> OR133/1
  Demux32/11 -> OR129/1
  Demux32/1 -> OR130/1
  Demux32/15 -> OR135/1
  Demux32/10 -> OR128/2
  Demux32/9 -> OR128/1
  Demux32/6 -> OR132/2
  Demux32/12 -> OR129/2
  Demux32/16 -> OR135/2
  Demux32/3 -> OR131/1
  Demux32/2 -> OR130/2
  Demux32/4 -> OR131/2
  Demux32/8 -> OR133/2
  DoorMotorCircuitFailure/1 -> Demux35/1
  DoorFailedToLock/1 -> Demux32/1
  DoorFailedToUnlock/1 -> Demux31/1
  DoorUnexpectedUnlocking/1 -> Demux30/1
  DCSRFailure/1 -> Demux29/1
  Demux33/14 -> OR18/2
  Demux33/5 -> OR16/1
  Demux33/13 -> OR18/1
  Demux33/7 -> OR17/1
  Demux33/11 -> OR21/1
  Demux33/1 -> OR22/1
  Demux33/15 -> OR19/1
  Demux33/10 -> OR20/2
  Demux33/9 -> OR20/1
  Demux33/6 -> OR16/2
  Demux33/12 -> OR21/2
  Demux33/16 -> OR19/2
  Demux33/3 -> OR23/1
  Demux33/2 -> OR22/2
  Demux33/4 -> OR23/2
  Demux33/8 -> OR17/2
  DoorLockedStatus/1 -> Demux33/1
  OR22/1 -> Data Type Conversion98/1
  OR23/1 -> Data Type Conversion99/1
  OR17/1 -> Data Type Conversion101/1
  OR16/1 -> Data Type Conversion100/1
  OR18/1 -> Data Type Conversion102/1
  OR19/1 -> Data Type Conversion103/1
  OR21/1 -> Data Type Conversion105/1
  OR20/1 -> Data Type Conversion104/1
  OR60/1 -> Data Type Conversion110/1
  OR61/1 -> Data Type Conversion111/1
  OR59/1 -> Data Type Conversion109/1
  OR58/1 -> Data Type Conversion108/1
  OR56/1 -> Data Type Conversion106/1
  OR57/1 -> Data Type Conversion107/1
  OR63/1 -> Data Type Conversion113/1
  OR62/1 -> Data Type Conversion112/1
  DoorOpenObstruction/1 -> Demux24/1
  Demux24/8 -> OR57/2
  Demux24/4 -> OR63/2
  Demux24/2 -> OR62/2
  Demux24/3 -> OR63/1
  Demux24/16 -> OR59/2
  Demux24/12 -> OR61/2
  Demux24/6 -> OR56/2
  Demux24/9 -> OR60/1
  Demux24/10 -> OR60/2
  Demux24/15 -> OR59/1
  Demux24/1 -> OR62/1
  Demux24/11 -> OR61/1
  Demux24/7 -> OR57/1
  Demux24/13 -> OR58/1
  Demux24/5 -> OR56/1
  Demux24/14 -> OR58/2
  OR52/1 -> Data Type Conversion118/1
  OR53/1 -> Data Type Conversion119/1
  OR51/1 -> Data Type Conversion117/1
  OR50/1 -> Data Type Conversion116/1
  OR48/1 -> Data Type Conversion114/1
  OR49/1 -> Data Type Conversion115/1
  OR55/1 -> Data Type Conversion121/1
  OR54/1 -> Data Type Conversion120/1
  DoorCloseObstruction/1 -> Demux22/1
  Demux22/8 -> OR49/2
  Demux22/4 -> OR55/2
  Demux22/2 -> OR54/2
  Demux22/3 -> OR55/1
  Demux22/16 -> OR51/2
  Demux22/12 -> OR53/2
  Demux22/6 -> OR48/2
  Demux22/9 -> OR52/1
  Demux22/10 -> OR52/2
  Demux22/15 -> OR51/1
  Demux22/1 -> OR54/1
  Demux22/11 -> OR53/1
  Demux22/7 -> OR49/1
  Demux22/13 -> OR50/1
  Demux22/5 -> OR48/1
  Demux22/14 -> OR50/2
  OR28/1 -> [DoorB1EmergencyReleased], Data Type Conversion126/1
  OR29/1 -> [DoorB2EmergencyReleased], Data Type Conversion127/1
  OR27/1 -> [DoorB4EmergencyReleased], Data Type Conversion125/1
  OR26/1 -> [DoorB3EmergencyReleased], Data Type Conversion124/1
  OR24/1 -> [DoorA3EmergencyReleased], Data Type Conversion122/1
  OR25/1 -> [DoorA4EmergencyReleased], Data Type Conversion123/1
  OR30/1 -> [DoorA1EmergencyReleased], Data Type Conversion128/1
  DoorEmergencyReleasedStatus/1 -> Demux2/1
  Demux2/8 -> OR25/2
  Demux2/4 -> OR31/2
  Demux2/2 -> OR30/2
  Demux2/3 -> OR31/1
  Demux2/16 -> OR27/2
  Demux2/12 -> OR29/2
  Demux2/6 -> OR24/2
  Demux2/9 -> OR28/1
  Demux2/10 -> OR28/2
  Demux2/15 -> OR27/1
  Demux2/1 -> OR30/1
  Demux2/11 -> OR29/1
  Demux2/7 -> OR25/1
  Demux2/13 -> OR26/1
  Demux2/5 -> OR24/1
  Demux2/14 -> OR26/2
  OR36/1 -> Data Type Conversion134/1
  OR37/1 -> Data Type Conversion135/1
  OR35/1 -> Data Type Conversion133/1
  OR34/1 -> Data Type Conversion132/1
  OR32/1 -> Data Type Conversion130/1
  OR33/1 -> Data Type Conversion131/1
  OR39/1 -> Data Type Conversion137/1
  OR38/1 -> Data Type Conversion136/1
  DoorFaultStatus/1 -> Demux3/1
  Demux3/8 -> OR33/2
  Demux3/4 -> OR39/2
  Demux3/2 -> OR38/2
  Demux3/3 -> OR39/1
  Demux3/16 -> OR35/2
  Demux3/12 -> OR37/2
  Demux3/6 -> OR32/2
  Demux3/9 -> OR36/1
  Demux3/10 -> OR36/2
  Demux3/15 -> OR35/1
  Demux3/1 -> OR38/1
  Demux3/11 -> OR37/1
  Demux3/7 -> OR33/1
  Demux3/13 -> OR34/1
  Demux3/5 -> OR32/1
  Demux3/14 -> OR34/2
  OR44/1 -> Data Type Conversion142/1
  OR45/1 -> Data Type Conversion143/1
  OR43/1 -> Data Type Conversion141/1
  OR42/1 -> Data Type Conversion140/1
  OR40/1 -> Data Type Conversion138/1
  OR41/1 -> Data Type Conversion139/1
  OR47/1 -> Data Type Conversion145/1
  OR46/1 -> Data Type Conversion144/1
  DoorIsolatedStatus/1 -> Demux4/1
  Demux4/8 -> OR41/2
  Demux4/4 -> OR47/2
  Demux4/2 -> OR46/2
  Demux4/3 -> OR47/1
  Demux4/16 -> OR43/2
  Demux4/12 -> OR45/2
  Demux4/6 -> OR40/2
  Demux4/9 -> OR44/1
  Demux4/10 -> OR44/2
  Demux4/15 -> OR43/1
  Demux4/1 -> OR46/1
  Demux4/11 -> OR45/1
  Demux4/7 -> OR41/1
  Demux4/13 -> OR42/1
  Demux4/5 -> OR40/1
  Demux4/14 -> OR42/2
  OR12/1 -> Data Type Conversion150/1
  OR13/1 -> Data Type Conversion151/1
  OR11/1 -> Data Type Conversion149/1
  OR10/1 -> Data Type Conversion148/1
  OR8/1 -> Data Type Conversion146/1
  OR9/1 -> Data Type Conversion147/1
  OR15/1 -> Data Type Conversion153/1
  OR14/1 -> Data Type Conversion152/1
  DoorOpenStatus/1 -> Demux1/1
  Demux1/8 -> OR9/2
  Demux1/4 -> OR15/2
  Demux1/2 -> OR14/2
  Demux1/3 -> OR15/1
  Demux1/16 -> OR11/2
  Demux1/12 -> OR13/2
  Demux1/6 -> OR8/2
  Demux1/9 -> OR12/1
  Demux1/10 -> OR12/2
  Demux1/15 -> OR11/1
  Demux1/1 -> OR14/1
  Demux1/11 -> OR13/1
  Demux1/7 -> OR9/1
  Demux1/13 -> OR10/1
  Demux1/5 -> OR8/1
  Demux1/14 -> OR10/2
  For Each Subsystem6/1(WireState1) -> Demux16/1
  For Each Subsystem6/2(WireState2) -> Demux15/1
  Vector Concatenate15/1 -> For Each Subsystem6/2(Source2)
  Vector Concatenate14/1 -> For Each Subsystem6/1(Source1)
  [Orientation] -> For Each Subsystem6/3(Orientation)
  Demux/1 -> Data Type Conversion1/1
  Demux/2 -> Data Type Conversion154/1
  Demux/3 -> Data Type Conversion155/1
  Demux/4 -> Data Type Conversion156/1
  Demux/5 -> Data Type Conversion157/1
  Demux/6 -> Data Type Conversion158/1
  Demux/7 -> Data Type Conversion159/1
  Demux/8 -> Data Type Conversion160/1
  DCUPower/1 -> Demux/1
  Data Type Conversion1/1 -> Vector Concatenate14/1
  Data Type Conversion154/1 -> Vector Concatenate14/2
  Data Type Conversion155/1 -> Vector Concatenate14/3
  Data Type Conversion156/1 -> Vector Concatenate14/4
  Data Type Conversion157/1 -> Vector Concatenate15/1
  Data Type Conversion158/1 -> Vector Concatenate15/2
  Data Type Conversion159/1 -> Vector Concatenate15/3
  Data Type Conversion160/1 -> Vector Concatenate15/4
  In Bus Element/1 -> OR142/1
  In Bus Element2/1 -> OR143/1
  In Bus Element3/1 -> OR136/1
  In Bus Element4/1 -> OR137/1
  In Bus Element5/1 -> OR140/1
  In Bus Element6/1 -> OR141/1
  In Bus Element7/1 -> OR138/1
  In Bus Element8/1 -> OR139/1
  OR142/1 -> SR Latch - Reset Priority/1
  OR143/1 -> SR Latch - Reset Priority1/1
  OR136/1 -> SR Latch - Reset Priority2/1
  OR137/1 -> SR Latch - Reset Priority3/1
  OR140/1 -> SR Latch - Reset Priority4/1
  OR141/1 -> SR Latch - Reset Priority5/1
  OR138/1 -> SR Latch - Reset Priority6/1
  OR139/1 -> SR Latch - Reset Priority7/1
  OR31/1 -> [DoorA2EmergencyReleased], Data Type Conversion129/1
  [DoorA4EmergencyReleased] -> Detect Decrease/1, OR137/2
  Detect Decrease/1 -> SR Latch - Reset Priority3/2
  Detect Decrease7/1 -> SR Latch - Reset Priority7/2
  Detect Decrease6/1 -> SR Latch - Reset Priority6/2
  Detect Decrease5/1 -> SR Latch - Reset Priority5/2
  Detect Decrease4/1 -> SR Latch - Reset Priority4/2
  [DoorA3EmergencyReleased] -> Detect Decrease1/1, OR136/2
  [DoorA2EmergencyReleased] -> Detect Decrease2/1, OR143/2
  [DoorA1EmergencyReleased] -> Detect Decrease3/1, OR142/2
  [DoorB1EmergencyReleased] -> Detect Decrease4/1, OR140/2
  [DoorB2EmergencyReleased] -> Detect Decrease5/1, OR141/2
  [DoorB3EmergencyReleased] -> Detect Decrease6/1, OR138/2
  [DoorB4EmergencyReleased] -> Detect Decrease7/1, OR139/2
  Detect Decrease1/1 -> SR Latch - Reset Priority2/2
  Detect Decrease2/1 -> SR Latch - Reset Priority1/2
  Detect Decrease3/1 -> SR Latch - Reset Priority/2
  SR Latch - Reset Priority7/1 -> Data Type Conversion168/1
  SR Latch - Reset Priority6/1 -> Data Type Conversion167/1
  SR Latch - Reset Priority5/1 -> Data Type Conversion166/1
  SR Latch - Reset Priority4/1 -> Data Type Conversion165/1
  SR Latch - Reset Priority3/1 -> Data Type Conversion164/1
  SR Latch - Reset Priority2/1 -> Data Type Conversion163/1
  SR Latch - Reset Priority1/1 -> Data Type Conversion162/1
  SR Latch - Reset Priority/1 -> Data Type Conversion161/1
  Data Type Conversion161/1 -> Bus Creator/162  "DoorA1LocalEED"
  Data Type Conversion162/1 -> Bus Creator/163  "DoorA2LocalEED"
  Data Type Conversion163/1 -> Bus Creator/164  "DoorA3LocalEED"
  Data Type Conversion164/1 -> Bus Creator/165  "DoorA4LocalEED"
  Data Type Conversion165/1 -> Bus Creator/166  "DoorB1LocalEED"
  Data Type Conversion166/1 -> Bus Creator/167  "DoorB2LocalEED"
  Data Type Conversion167/1 -> Bus Creator/168  "DoorB3LocalEED"
  Data Type Conversion168/1 -> Bus Creator/169  "DoorB4LocalEED"

== system TCMSSystem/TCMSSystemPerVehicle/EnabledTCMSVehicle/TCMSElectrical/ElectricalControl/Doors/Subsystem4 ==
  note: MMRBEM-3941
  LeftDoorsEnable : Inport
  AllLeftDoorsClosed : Inport  Port=2
  ATCLeftDoorCloseAuth : Inport  Port=3
  LeftHoldDooorClose : Inport  Port=4
  Logical Operator : Logic  AllPortsSameDT=off  OutDataTypeStr=boolean
  NOT1 : Logic  Operator=NOT  AllPortsSameDT=off  OutDataTypeStr=boolean
  NOT2 : Logic  Operator=NOT  AllPortsSameDT=off  OutDataTypeStr=boolean
  Pulse Generator1 : DiscretePulseGenerator  PulseType=Time based  Period=1  PulseWidth=50
  Pulse Generator2 : DiscretePulseGenerator  PulseType=Time based  Period=1  PulseWidth=50
  SteadyOFF : Constant  Value=0
  SteadyON : Constant
  SteadyON. : Constant
  Switch{,1..4} (5 alike) : Switch  Criteria=u2 > Threshold
  LeftDoorsAuth&Closed : Outport
  LeftDoorsAuth&Opened : Outport  Port=2
  wires:
  AllLeftDoorsClosed/1 -> NOT1/1, Switch3/2, Switch/3, Switch1/2
  Logical Operator/1 -> Switch/2, Switch2/2
  NOT1/1 -> Switch2/3
  Switch3/1 -> Switch2/1
  SteadyON/1 -> Switch1/1
  Pulse Generator2/1 -> Switch4/1
  Pulse Generator1/1 -> Switch3/1
  SteadyON./1 -> Switch3/3
  Switch1/1 -> Switch/1
  Switch2/1 -> LeftDoorsAuth&Opened/1  "LeftDoorsAuth&Opened"
  Switch/1 -> LeftDoorsAuth&Closed/1  "LeftDoorsAuth&Closed"
  SteadyOFF/1 -> Switch4/3
  Switch4/1 -> Switch1/3
  ATCLeftDoorCloseAuth/1 -> Switch4/2
  LeftDoorsEnable/1 -> Logical Operator/1
  LeftHoldDooorClose/1 -> NOT2/1
  NOT2/1 -> Logical Operator/2

== system TCMSSystem/TCMSSystemPerVehicle/EnabledTCMSVehicle/TCMSElectrical/ElectricalControl/Doors/Subsystem5 ==
  In1 : Inport  Partition=on  PartitionDimension=1  PartitionWidth=1  PartitionOffset=0
  Bus Selector : BusSelector  OutputSignals=DoorReleasedAuthorisedToOpenStatus
  For Each : ForEach  DisableCoverage=on
  DoorAuthorized : Outport  ConcatenationDimension=1
  wires:
  In1/1 -> Bus Selector/1
  Bus Selector/1 -> DoorAuthorized/1  "<DoorReleasedAuthorisedToOpenStatus>"

== system TCMSSystem/TCMSSystemPerVehicle/EnabledTCMSVehicle/TCMSElectrical/ElectricalControl/Doors/Subsystem6 ==
  note: MMRBEM-3941
  RightDoorsEnable : Inport
  AllRightDoorsClosed : Inport  Port=2
  ATCRightDoorCloseAuth : Inport  Port=3
  RightHoldDooorClose : Inport  Port=4
  Logical Operator : Logic  AllPortsSameDT=off  OutDataTypeStr=boolean
  NOT1 : Logic  Operator=NOT  AllPortsSameDT=off  OutDataTypeStr=boolean
  NOT2 : Logic  Operator=NOT  AllPortsSameDT=off  OutDataTypeStr=boolean
  Pulse Generator1 : DiscretePulseGenerator  PulseType=Time based  Period=1  PulseWidth=50
  Pulse Generator2 : DiscretePulseGenerator  PulseType=Time based  Period=1  PulseWidth=50
  SteadyOFF : Constant  Value=0
  SteadyON : Constant
  SteadyON. : Constant
  Switch{,1..4} (5 alike) : Switch  Criteria=u2 > Threshold
  RightDoorsAuth&Closed : Outport
  RightDoorsAuth&Opened : Outport  Port=2
  wires:
  Switch/1 -> RightDoorsAuth&Closed/1  "RightDoorsAuth&Closed"
  Switch2/1 -> RightDoorsAuth&Opened/1  "RightDoorsAuth&Opened"
  Switch1/1 -> Switch/1
  SteadyON./1 -> Switch3/3
  Pulse Generator1/1 -> Switch3/1
  Switch4/1 -> Switch1/3
  SteadyON/1 -> Switch1/1
  Switch3/1 -> Switch2/1
  NOT1/1 -> Switch2/3
  Logical Operator/1 -> Switch2/2, Switch/2
  AllRightDoorsClosed/1 -> Switch1/2, Switch/3, Switch3/2, NOT1/1
  Pulse Generator2/1 -> Switch4/1
  SteadyOFF/1 -> Switch4/3
  ATCRightDoorCloseAuth/1 -> Switch4/2
  NOT2/1 -> Logical Operator/2
  RightDoorsEnable/1 -> Logical Operator/1
  RightHoldDooorClose/1 -> NOT2/1

== system TCMSSystem/TCMSSystemPerVehicle/EnabledTCMSVehicle/TCMSElectrical/ElectricalDisplay/EnableToRunScreen/CabUnitDisplay ==
  ElectricalSignals : Inport
  WireStates : Inport  Port=2
  CBTC : Inport  Port=3
  Bus Selector1 : BusSelector  OutputSignals=CabActive
  CabActiveUnitDisplay : Subsystem  TreatAsAtomicUnit=on
  CabInActiveUnitDisplay : Subsystem  TreatAsAtomicUnit=on
  Data Type Conversion : DataTypeConversion  OutDataTypeStr=uint32
  If : If
  Merge : Merge
  CabUnitDisplay : Outport
  wires:
  Merge/1 -> CabUnitDisplay/1
  CabInActiveUnitDisplay/1(Out1) -> Merge/2
  CabActiveUnitDisplay/1(Out1) -> Merge/1
  If/2 -> CabInActiveUnitDisplay/Action
  If/1 -> CabActiveUnitDisplay/Action
  Data Type Conversion/1 -> If/1
  Bus Selector1/1 -> Data Type Conversion/1  "<CabActive>"
  ElectricalSignals/1 -> CabActiveUnitDisplay/1(ElectricalSignals), Bus Selector1/1
  WireStates/1 -> CabActiveUnitDisplay/2(WireStates)
  CBTC/1 -> CabActiveUnitDisplay/3(CBTC)

== system TCMSSystem/TCMSSystemPerVehicle/EnabledTCMSVehicle/TCMSElectrical/ElectricalDisplay/OperatingandHeaderScreen/CabUnitDisplay ==
  TCMSConfig : Inport
  ElectricalSignals : Inport  Port=2
  Bus Selector1 : BusSelector  OutputSignals=HasCab
  CabActiveUnitDisplay : Subsystem  TreatAsAtomicUnit=on
  CabInActiveUnitDisplay : Subsystem  TreatAsAtomicUnit=on
  Data Type Conversion : DataTypeConversion  OutDataTypeStr=uint32
  If : If
  Merge : Merge
  CabUnitDisplay : Outport
  wires:
  Merge/1 -> CabUnitDisplay/1
  CabInActiveUnitDisplay/1(Out1) -> Merge/2
  CabActiveUnitDisplay/1(Out1) -> Merge/1
  If/2 -> CabInActiveUnitDisplay/Action
  If/1 -> CabActiveUnitDisplay/Action
  Data Type Conversion/1 -> If/1
  Bus Selector1/1 -> Data Type Conversion/1  "<HasCab>"
  TCMSConfig/1 -> Bus Selector1/1
  ElectricalSignals/1 -> CabActiveUnitDisplay/1(ElectricalSignals)

== system TCMSSystem/TCMSSystemPerVehicle/EnabledTCMSVehicle/TCMSElectrical/ElectricalDisplay/OperatingandHeaderScreen/Subsystem ==
  note: Motoring
      | AND
      | No Zerospeed
  note: Motoring
      | AND
      | Zerospeed
  note: Not Motoring
      | AND
      | (Braking
      | OR
      | Zerospeed)
  In Bus Element : Inport  PortName=ElectricalSignals  Element=MotorTrainLine
  In Bus Element1 : Inport  PortName=ElectricalSignals  Element=BrakeTrainLine
  In Bus Element2 : Inport  PortName=ElectricalSignals  Element=FSB1Line
  In Bus Element3 : Inport  PortName=ElectricalSignals  Element=FSB2Line
  In Bus Element4 : Inport  PortName=ElectricalSignals  Element=EB1Line
  In Bus Element5 : Inport  PortName=ElectricalSignals  Element=EB2Line
  In Bus Element6 : Inport  PortName=ElectricalSignals  Element=ZeroSpeed
  In Bus Element7 : Inport  PortName=ElectricalSignals  Element=Speedometer
  Compare To Zero1 : simulink/Logic and Bit Operations/Compare To Zero  relop=>  OutDataTypeStr=boolean
  If : If  NumInputs=3  IfExpression=u1 & ~u3  ElseIfExpressions=u1 & u3, ~u1 & (u2 | u3)  ShowElse=off
  If Action Subsystem : Subsystem  TreatAsAtomicUnit=on
  If Action Subsystem1 : Subsystem  TreatAsAtomicUnit=on
  If Action Subsystem2 : Subsystem  TreatAsAtomicUnit=on
  Merge : Merge  Inputs=3
  OR : Logic  Operator=NAND  Inputs=5  AllPortsSameDT=off  OutDataTypeStr=boolean
  OR1 : Logic  Operator=OR  AllPortsSameDT=off  OutDataTypeStr=boolean
  OperationalMode : Outport
  wires:
  If/1 -> If Action Subsystem/Action  "RUNNING"
  If/2 -> If Action Subsystem1/Action  "RUN READY"
  If/3 -> If Action Subsystem2/Action  "RUN NOT READY"
  Merge/1 -> OperationalMode/1
  If Action Subsystem1/1(Out1) -> Merge/2
  If Action Subsystem2/1(Out1) -> Merge/3
  If Action Subsystem/1(Out1) -> Merge/1
  OR1/1 -> If/1  "Motoring"
  In Bus Element1/1 -> OR/1
  In Bus Element2/1 -> OR/2
  In Bus Element3/1 -> OR/3
  In Bus Element4/1 -> OR/4
  In Bus Element5/1 -> OR/5
  OR/1 -> If/2  "Braking"
  In Bus Element6/1 -> If/3
  In Bus Element/1 -> OR1/1  "Motoring"
  In Bus Element7/1 -> Compare To Zero1/1
  Compare To Zero1/1 -> OR1/2

== system TCMSSystem/TCMSSystemPerVehicle/EnabledTCMSVehicle/TCMSElectrical/ElectricalDisplay/OperatingandHeaderScreen/Subsystem1 ==
  DrivingMode : Inport
  CommonConfig : Inport  Port=2
  RescureModeCondition : Inport  Port=3
  CommonVehicleConfig : Inport  Port=4
  Add Constant : Bias  Bias=-1
  Bus Selector : BusSelector  OutputSignals=Orientation
  Bus Selector1 : BusSelector  OutputSignals=HasCab
  CouplerNumber : Selector  InputPortWidth=2  IndexOptions=Index vector (dialog)  Indices=2  OutputSizes=1
  CouplerNumber1 : Selector  InputPortWidth=2  IndexOptions=Index vector (dialog)  Indices=1  OutputSizes=1
  Logical Operator1 : Logic  AllPortsSameDT=off  OutDataTypeStr=boolean
  Logical Operator2 : Logic  AllPortsSameDT=off  OutDataTypeStr=boolean
  OR : Logic  Operator=OR  AllPortsSameDT=off  OutDataTypeStr=boolean
  RMF1 : simulink/Logic and Bit Operations/Compare To Constant  relop===  const=3  OutDataTypeStr=boolean
  RMR1 : simulink/Logic and Bit Operations/Compare To Constant  relop===  const=1  OutDataTypeStr=boolean
  Switch : Switch  Criteria=u2 > Threshold
  RescueMode : Outport
  wires:
  Add Constant/1 -> Switch/2
  Bus Selector/1 -> Add Constant/1  "<Orientation>"
  Switch/1 -> Logical Operator2/2
  Logical Operator1/1 -> CouplerNumber1/1, CouplerNumber/1
  CommonVehicleConfig/1 -> Bus Selector/1
  CouplerNumber1/1 -> Switch/3
  CouplerNumber/1 -> Switch/1
  RMR1/1 -> OR/2
  OR/1 -> Logical Operator2/1
  RMF1/1 -> OR/1
  Logical Operator2/1 -> RescueMode/1
  DrivingMode/1 -> RMF1/1, RMR1/1
  CommonConfig/1 -> Bus Selector1/1
  Bus Selector1/1 -> Logical Operator1/1  "<HasCab>"
  RescureModeCondition/1 -> Logical Operator1/2

== system TCMSSystem/TCMSSystemPerVehicle/EnabledTCMSVehicle/TCMSPantograph/PantographDisplay/CabUnitDisplay/CabActiveUnitDisplay ==
  In Bus Element : Inport  PortName=ElectricalSignals  Element=PantoLowered
  In Bus Element1 : Inport  PortName=ElectricalSignals  Element=PantoRaised
  In Bus Element2 : Inport  PortName=ElectricalSignals  Element=PantoPowerDetected
  Action Port : ActionPort  ActionPortLabel=if(u1 > 0)
  Bus Creator : BusCreator  Inputs=3
  Data Type Conversion : DataTypeConversion  OutDataTypeStr=double
  Data Type Conversion1 : DataTypeConversion  OutDataTypeStr=double
  Data Type Conversion2 : DataTypeConversion  OutDataTypeStr=double
  Out1 : Outport
  wires:
  Bus Creator/1 -> Out1/1
  In Bus Element1/1 -> Data Type Conversion/1
  In Bus Element2/1 -> Data Type Conversion2/1
  In Bus Element/1 -> Data Type Conversion1/1
  Data Type Conversion/1 -> Bus Creator/1  "UnitAtLeastOnePantoUp"
  Data Type Conversion1/1 -> Bus Creator/2  "UnitAllPantoDown"
  Data Type Conversion2/1 -> Bus Creator/3  "UnitPantoPowerDetected"

== system TCMSSystem/TCMSSystemPerVehicle/EnabledTCMSVehicle/TCMSPantograph/PantographDisplay/CabUnitDisplay/CabInActiveUnitDisplay ==
  Action Port : ActionPort  ActionPortLabel=else
  Bus Creator : BusCreator  Inputs=3
  Constant : Constant  Value=0
  Constant1 : Constant  Value=0
  Constant2 : Constant  Value=0
  Out1 : Outport
  wires:
  Bus Creator/1 -> Out1/1
  Constant/1 -> Bus Creator/1  "UnitAtLeastOnePantoUp"
  Constant1/1 -> Bus Creator/2  "UnitAllPantoDown"
  Constant2/1 -> Bus Creator/3  "UnitPantoPowerDetected"

== system TCMSSystem/TCMSSystemPerVehicle/EnabledTCMSVehicle/TCMSPneumatics/PneumaticsDisplay/CabUnitDisplay/CabActiveUnitDisplay ==
  In Bus Element5 : Inport  PortName=ElectricalSignals  Element=ParkBrakeApplication
  In Bus Element : Inport  PortName=ElectricalSignals  Element=ServiceBrakesReleased
  In Bus Element1 : Inport  PortName=ElectricalSignals  Element=ParkBrakesReleased
  Action Port : ActionPort  ActionPortLabel=if(u1 > 0)
  Bus Creator : BusCreator  Inputs=4
  Data Type Conversion{,1..3} (4 alike) : DataTypeConversion  OutDataTypeStr=double
  NOT : Logic  Operator=NOT  AllPortsSameDT=off  OutDataTypeStr=boolean
  Out1 : Outport
  wires:
  Data Type Conversion2/1 -> Bus Creator/3  "AllParkBrakesReleased"
  Data Type Conversion1/1 -> Bus Creator/2  "ServiceBrakesApplied"
  Data Type Conversion/1 -> Bus Creator/1  "AllServiceBrakesReleased"
  Bus Creator/1 -> Out1/1
  In Bus Element/1 -> NOT/1, Data Type Conversion/1
  Data Type Conversion3/1 -> Bus Creator/4  "ParkBrakesApplied"
  In Bus Element1/1 -> Data Type Conversion2/1
  In Bus Element5/1 -> Data Type Conversion3/1
  NOT/1 -> Data Type Conversion1/1

== system TCMSSystem/TCMSSystemPerVehicle/EnabledTCMSVehicle/TCMSPneumatics/PneumaticsDisplay/CabUnitDisplay/CabInActiveUnitDisplay ==
  Action Port : ActionPort  ActionPortLabel=else
  Bus Creator : BusCreator  Inputs=4
  Constant{,1..3} (4 alike) : Constant  Value=0
  Out1 : Outport
  wires:
  Bus Creator/1 -> Out1/1
  Constant3/1 -> Bus Creator/4  "ParkBrakesApplied"
  Constant1/1 -> Bus Creator/2  "ServiceBrakesApplied"
  Constant2/1 -> Bus Creator/3  "AllParkBrakesReleased"
  Constant/1 -> Bus Creator/1  "AllServiceBrakesReleased"
